simulink model "h_sezione"  (R2023a)
settings: Solver=VariableStepAuto  StartTime=0.0  StopTime=500.0  RelTol=1e-3
undefined symbols (not defined in the file or in its folder): h_limite, r_grande, r_piccolo, theta_grande, theta_piccolo
libraries: simulink x1
settings Model: Creator=pmong  LastModifiedBy=pmong

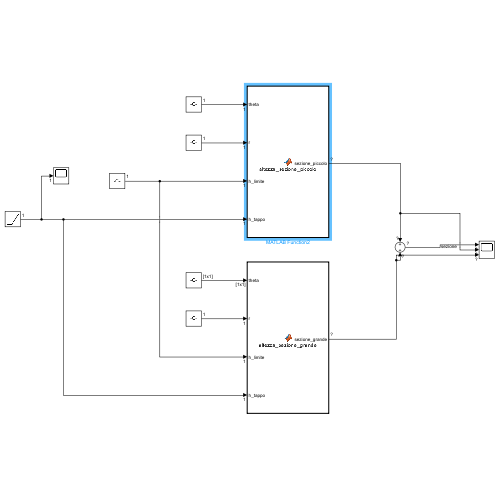
[thumbnail: Simulink's stored preview of the top-level diagram]
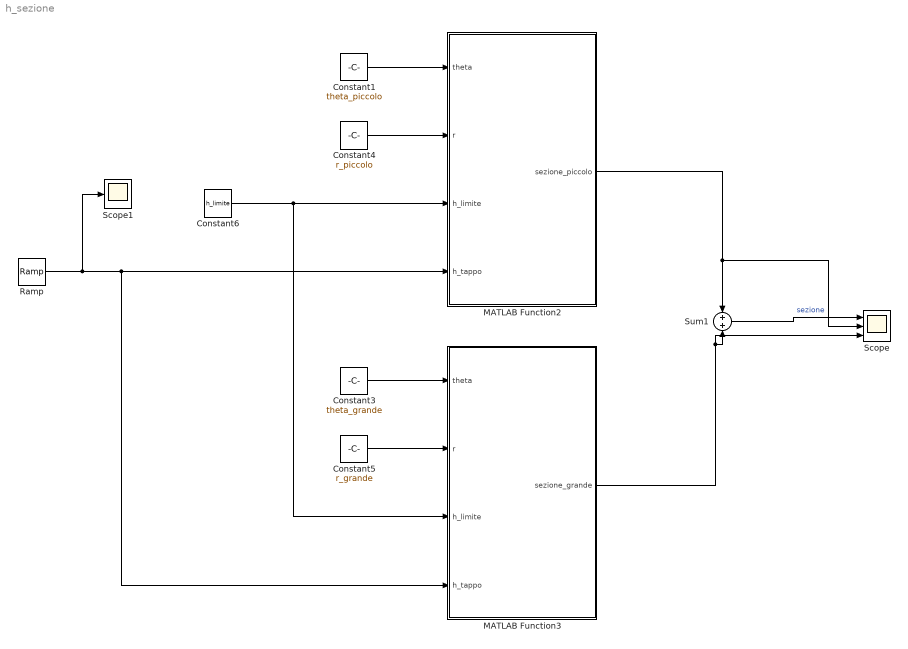
== system h_sezione ==
  Constant1 : Constant  Value=theta_piccolo
  Constant3 : Constant  Value=theta_grande  VectorParams1D=off
  Constant4 : Constant  Value=r_piccolo
  Constant5 : Constant  Value=r_grande
  Constant6 : Constant  Value=h_limite
  MATLAB Function2 : MATLAB Function  TreatAsAtomicUnit=on
  MATLAB Function3 : MATLAB Function  TreatAsAtomicUnit=on
  Ramp : simulink/Sources/Ramp  slope=0.0001  start=50  InitialOutput=0
  Scope : Scope  NumInputPorts=3
  Scope1 : Scope
  Sum1 : Sum
  wires:
  Constant1/1 -> MATLAB Function2/1(theta)
  MATLAB Function3/1(sezione_grande) -> Scope/3, Sum1/2
  Constant6/1 -> MATLAB Function3/3(h_limite), MATLAB Function2/3(h_limite)
  Constant4/1 -> MATLAB Function2/2(r)
  MATLAB Function2/1(sezione_piccolo) -> Scope/2, Sum1/1
  Sum1/1 -> Scope/1  "sezione"
  Constant5/1 -> MATLAB Function3/2(r)
  Ramp/1 -> Scope1/1, MATLAB Function3/4(h_tappo), MATLAB Function2/4(h_tappo)
  Constant3/1 -> MATLAB Function3/1(theta)

== matlab function h_sezione/MATLAB Function2 ==
  data: theta input; sezione_piccolo output; r input; h_limite input; h_tappo input
function sezione_piccolo = altezza_sezione_piccolo(theta, r, h_limite, h_tappo)

if h_tappo >= h_limite
    h_tappo = h_limite;     % questa sezione non si apre di più quando si apre il grande
end


m = tan(theta);
y0 = r * m;

xg = r;
yg = y0;

a = sin(pi/2 - theta) * h_tappo;

xr = r - a * sin(theta);
yr = y0+a*cos(theta);


sezione_piccolo = pi * (xg - xr) * a;

== matlab function h_sezione/MATLAB Function3 ==
  data: theta input; sezione_grande output; r input; h_limite input; h_tappo input
function sezione_grande = altezza_sezione_grande(theta, r, h_limite, h_tappo)

if h_tappo < h_limite
    h_tappo = 0;    
else
    h_tappo = h_tappo - h_limite;
end

m = tan(theta);
y0 = r * m;

xg = r;
yg = y0;

a = sin(pi/2 - theta) * h_tappo;

xr = r - a * sin(theta);
yr = y0+a*cos(theta);


sezione_grande = pi * (xg - xr) * a;
